simulink model "LinearModel_RudderActuator2"  (R2015a)
settings: Solver=ode23s  StartTime=0.0  StopTime=5  FixedStep=1e-4  RelTol=1e-3
values from neighbouring files (symbols this model uses):
  StateControl =     [StateControl.mat]
undefined symbols (not defined in the file or in its folder): EHSV_Step
settings Model: Creator=HERIC  LastModifiedBy=Pedro H
settings OptimizationCC: ExpressionDepthLimit=2147483647
settings DebuggingCC: UnderspecifiedInitializationDetection=Classic  MergeDetectMultiDrivingBlocksExec=none  SolverPrmCheckMsg=warning  StateNameClashWarn=warning

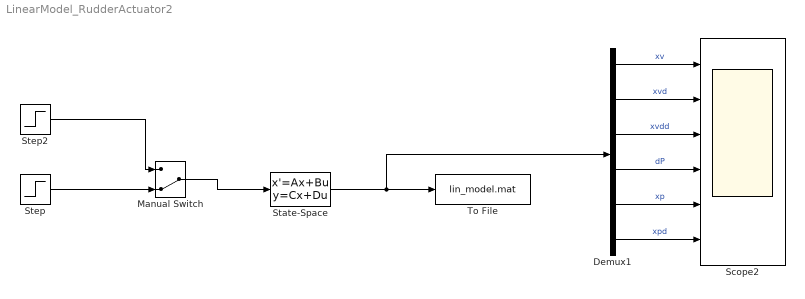
== system LinearModel_RudderActuator2 ==
  Demux1 : Demux  Outputs=6
  Manual Switch : ManualSwitch  CurrentSetting=0
  Scope2 : Scope  NumInputPorts=6
      settings: TimeRange=1.515675675675676  YMin=-5.9091e-26~-400000~0~-6.08696e-06~-1.15432e-20~-5e-06  YMax=0.0671053~200000~300000~3.3913e-05~0.04~5e-06  SaveName=ScopeData2
  State-Space : StateSpace  A=StateControl.A  B=StateControl.B  C=eye(6)  D=zeros(6,1)  X0=StateControl.X0
  Step : Step  Time=EHSV_Step.time  Before=EHSV_Step.initial  After=EHSV_Step.final
  Step2 : Step  Time=0.5  After=8
  To File : ToFile  Filename=lin_model.mat  MatrixName=states_lin  SaveFormat=Timeseries
  wires:
  Step/1 -> Manual Switch/2
  State-Space/1 -> Demux1/1, To File/1
  Manual Switch/1 -> State-Space/1
  Step2/1 -> Manual Switch/1
  Demux1/5 -> Scope2/5  "xp"
  Demux1/4 -> Scope2/4  "dP"
  Demux1/3 -> Scope2/3  "xvdd"
  Demux1/1 -> Scope2/1  "xv"
  Demux1/2 -> Scope2/2  "xvd"
  Demux1/6 -> Scope2/6  "xpd"
